simulink model "untitled"  (R2014a)
settings: Solver=ode45  StartTime=0.0  StopTime=10.0  RelTol=1e-3
libraries: arduino_io_lib x4, simulink x1
settings Model: Creator=omar_  LastModifiedBy=omar_

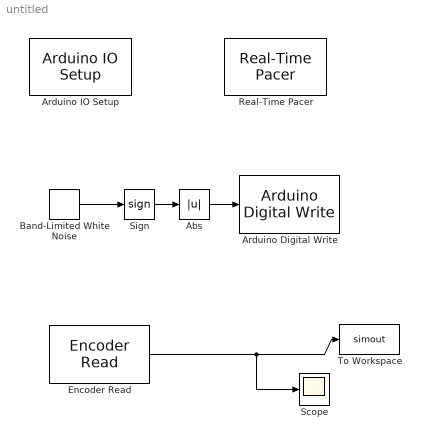
== system untitled ==
  Abs : Abs
  Arduino Digital Write : arduino_io_lib/Arduino Digital Write  arduinoVar=Temporary arduino variable: Arduino1  arduinoPin=4  T=-1
  Arduino IO Setup : arduino_io_lib/Arduino IO Setup  Priority=3  arduinoVar=Temporary arduino variable: Arduino1  workspaceVarName=a  comPort=COM12
  Band-Limited White Noise : simulink/Sources/Band-Limited White Noise  Cov=[0.1]  Ts=0.1  seed=[23341]
  Encoder Read : arduino_io_lib/Encoder Read  arduinoVar=Temporary arduino variable: Arduino1  encNum=1  pinA=3  pinB=2  DbDl=0  T=0.2
  Real-Time Pacer : arduino_io_lib/Real-Time Pacer  simTimePerRealTime=1
  Scope : Scope
  Sign : Signum
  To Workspace : ToWorkspace  VariableName=simout  SaveFormat=Timeseries  SampleTime=-1
  wires:
  Band-Limited White Noise/1 -> Sign/1
  Encoder Read/1 -> Scope/1, To Workspace/1
  Sign/1 -> Abs/1
  Abs/1 -> Arduino Digital Write/1
